simulink model "ControlTheoryHW3Q1 (1)"  (R2024a)
settings: Solver=VariableStepAuto  StartTime=0.0  StopTime=10.0  RelTol=1e-3

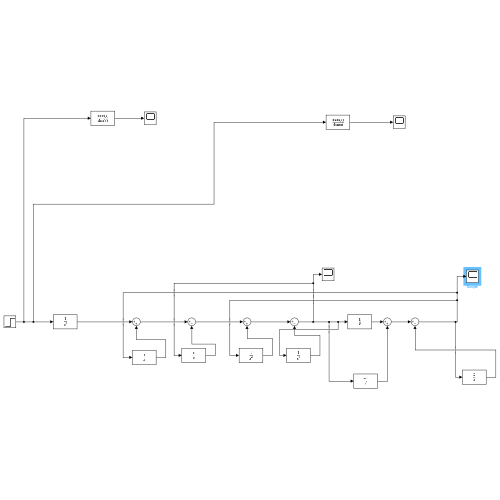
[thumbnail: Simulink's stored preview of the top-level diagram]
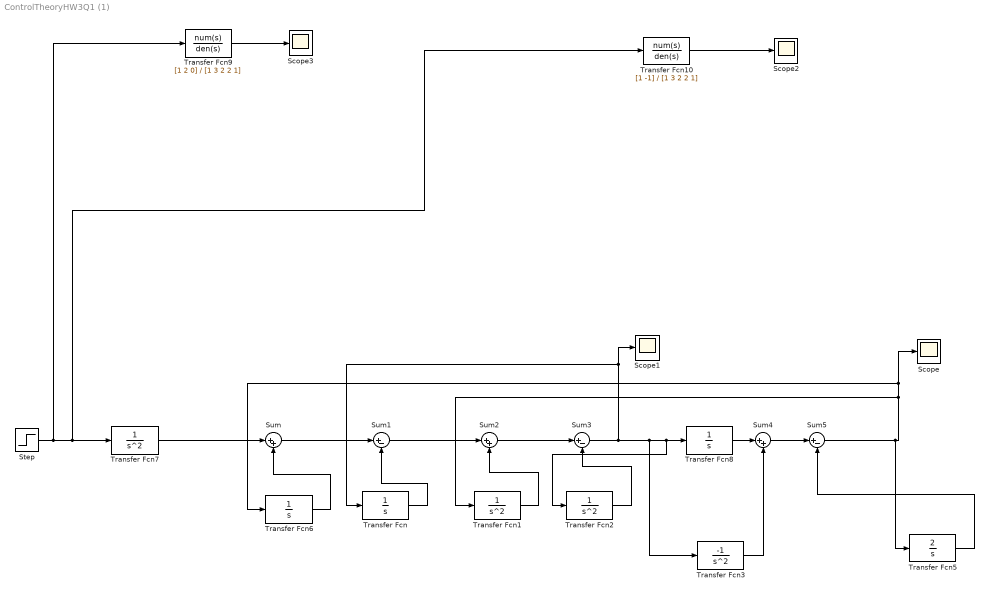
== system ControlTheoryHW3Q1 (1) ==
  Scope{,1..3} (4 alike) : Scope
  Step : Step  SampleTime=0
  Sum : Sum  Inputs=|++
  Sum1 : Sum  Inputs=|+-
  Sum2 : Sum  Inputs=|++
  Sum3 : Sum  Inputs=|+-
  Sum4 : Sum  Inputs=|++
  Sum5 : Sum  Inputs=|+-
  Transfer Fcn : TransferFcn  Denominator=[1 0]
  Transfer Fcn1 : TransferFcn  Denominator=[1 0 0]
  Transfer Fcn10 : TransferFcn  Numerator=[1 -1]  Denominator=[1 3 2 2 1]
  Transfer Fcn2 : TransferFcn  Denominator=[1 0 0]
  Transfer Fcn3 : TransferFcn  Numerator=[-1]  Denominator=[1 0 0]
  Transfer Fcn5 : TransferFcn  Numerator=[2]  Denominator=[1 0]
  Transfer Fcn6 : TransferFcn  Denominator=[1 0]
  Transfer Fcn7 : TransferFcn  Denominator=[1 0 0]
  Transfer Fcn8 : TransferFcn  Denominator=[1 0]
  Transfer Fcn9 : TransferFcn  Numerator=[1 2 0]  Denominator=[1 3 2 2 1]
  wires:
  Step/1 -> Transfer Fcn9/1, Transfer Fcn10/1, Transfer Fcn7/1
  Transfer Fcn7/1 -> Sum/1
  Sum/1 -> Sum1/1
  Sum1/1 -> Sum2/1
  Sum2/1 -> Sum3/1
  Sum3/1 -> Scope1/1, Transfer Fcn/1, Transfer Fcn3/1, Transfer Fcn2/1, Transfer Fcn8/1
  Transfer Fcn6/1 -> Sum/2
  Transfer Fcn/1 -> Sum1/2
  Transfer Fcn1/1 -> Sum2/2
  Transfer Fcn2/1 -> Sum3/2
  Transfer Fcn8/1 -> Sum4/1
  Sum4/1 -> Sum5/1
  Transfer Fcn3/1 -> Sum4/2
  Sum5/1 -> Transfer Fcn5/1, Transfer Fcn1/1, Transfer Fcn6/1, Scope/1
  Transfer Fcn9/1 -> Scope3/1
  Transfer Fcn10/1 -> Scope2/1
  Transfer Fcn5/1 -> Sum5/2
